simulink model "combined_model_withAC_2023"  (R2023a)
settings: Solver=VariableStepAuto  StartTime=0.0  StopTime=5  RelTol=1e-3
model workspace (MAT data in the model file):
  C = 0.00044
  L = 0.00025
undefined symbols (not defined in the file): C_phi, Ls, poles, R_load, Rs
libraries: spsDiodeLib x7, spsSeriesRLCBranchLib x6, spsVoltageMeasurementLib x5, spsMosfetLib x5, spsControlledVoltageSourceLib x3, simulink x3, spsCurrentMeasurementLib x2, spsParallelRLCBranchLib x2, spsGroundLib x1, spsParallelRLCLoadLib x1, spsVariableCapacitorLib x1, spspowerguiLib x1
settings Model: Creator=maarten  LastModifiedBy=maarten

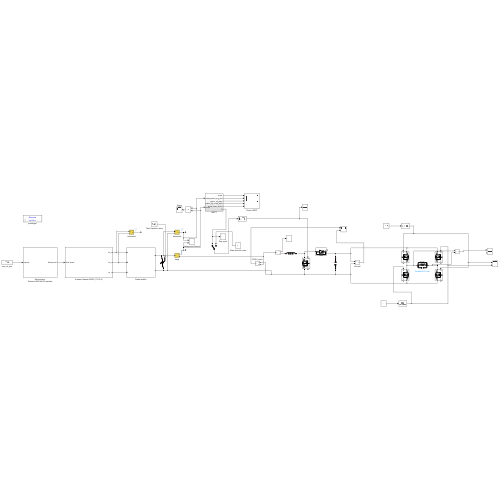
[thumbnail: Simulink's stored preview of the top-level diagram]
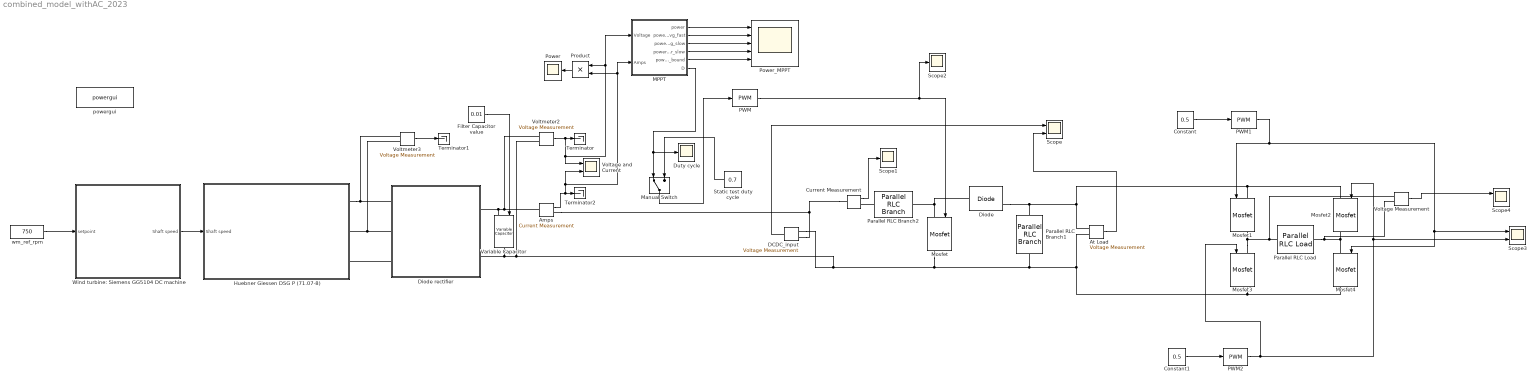
== system combined_model_withAC_2023 ==
  Amps : spsCurrentMeasurementLib/Current Measurement  PhasorSimulation=off  OutputType=Complex  PSBequivalent=0
  At Load : spsVoltageMeasurementLib/Voltage Measurement  PhasorSimulation=off  OutputType=Complex  PSBequivalent=0
  Constant : Constant  Value=0.5
  Constant1 : Constant  Value=0.5
  Current Measurement : spsCurrentMeasurementLib/Current Measurement  PhasorSimulation=off  OutputType=Complex  PSBequivalent=0
  DCDC_input : spsVoltageMeasurementLib/Voltage Measurement  PhasorSimulation=off  OutputType=Complex  PSBequivalent=0
  Diode : spsDiodeLib/Diode  Ron=0.001  Lon=0  Vf=0.8  IC=0  UseSnubber=0  Rs=500  Cs=250e-9  Measurements=on
  Diode rectifier : Subsystem
  Duty cycle : Scope
  Filter Capacitor value : Constant  Value=0.01
  "Huebner Giessen DSG P (71.07-8) " : Subsystem
  MPPT : Subsystem
  Manual Switch : ManualSwitch
  Mosfet{,1..4} (5 alike) : spsMosfetLib/Mosfet  Ron=0.1  Lon=0  Rd=0.01  Vfd=0  IC=0  Rs=1e5  Cs=inf  Measurements=on
  PWM : simulink/Discontinuities/PWM  DisableCoverage=on  Period=0.0001  InitialDelay=0  DisallowZeroDutyCycle=off  RunAtFixedTimeIntervals=off  SampleTime=0.1
  PWM1 : simulink/Discontinuities/PWM  DisableCoverage=on  Period=0.0005  InitialDelay=0  DisallowZeroDutyCycle=off  RunAtFixedTimeIntervals=off  SampleTime=0.1
  PWM2 : simulink/Discontinuities/PWM  DisableCoverage=on  Period=0.0005  InitialDelay=0.0005/2  DisallowZeroDutyCycle=off  RunAtFixedTimeIntervals=off  SampleTime=0.1
  Parallel RLC Branch1 : spsParallelRLCBranchLib/Parallel RLC Branch  LConnTagsString=a  RConnTagsString=__new0  BranchType=C  Resistance=R_load  Inductance=1e-3  SetiL0=off  InitialCurrent=0  Capacitance=C  Setx0=off  InitialVoltage=0  Measurements=None
  Parallel RLC Branch2 : spsParallelRLCBranchLib/Parallel RLC Branch  LConnTagsString=a  RConnTagsString=__new0  BranchType=L  Resistance=R_load  Inductance=L  SetiL0=off  InitialCurrent=0  Capacitance=C  Setx0=off  InitialVoltage=0  Measurements=None
  Parallel RLC Load : spsParallelRLCLoadLib/Parallel RLC Load  LConnTagsString=a  RConnTagsString=__new0  NominalVoltage=1000  NominalFrequency=60  ActivePower=10e3  InductivePower=100  CapacitivePower=100  Setx0=off  InitialVoltage=0  SetiL0=off  InitialCurrent=0  Measurements=None  LoadType=constant Z
      settings: AttributesFormatString=\n  LibrarySourceBlock=sps_lib/Passives/Parallel RLC Load
  Power : Scope
  Power_MPPT : Scope  NumInputPorts=5
  Product : Product
  Scope : Scope  NumInputPorts=2
  Scope1 : Scope
  Scope2 : Scope
  Scope3 : Scope  NumInputPorts=2
  Scope4 : Scope  NumInputPorts=2
  Static test duty cycle : Constant  Value=0.7
  Terminator : Terminator
  Terminator1 : Terminator
  Terminator2 : Terminator
  Variable Capacitor : spsVariableCapacitorLib/Variable Capacitor  methode=Backward Euler  Cabsmin=1e-9  Initialize=off  vC0=0  C0=1e-6  iC0=0
      settings: LibrarySourceBlock=sps_lib/Passives/Variable Capacitor
  Voltage Measurement : spsVoltageMeasurementLib/Voltage Measurement  PhasorSimulation=off  OutputType=Complex  PSBequivalent=0
  Voltage and Current : Scope  NumInputPorts=2
  Voltmeter2 : spsVoltageMeasurementLib/Voltage Measurement  PhasorSimulation=off  OutputType=Complex  PSBequivalent=0
  Voltmeter3 : spsVoltageMeasurementLib/Voltage Measurement  PhasorSimulation=off  OutputType=Complex  PSBequivalent=0
  "Wind turbine: Siemens GG5104 DC machine " : Subsystem
  powergui : spspowerguiLib/powergui  Priority=1  SimulationMode=Discrete  SampleTime=1e-6  frequency=60  Iterations=50  frequencyindice=0  Pbase=100e6  ErrMax=1e-4  UnitsV=kV  UnitsW=MW  buscounter=0  FunctionMessages=off  echomessages=off  EnableUseOfTLC=off  CurrentSourceSwitches=off  DisableSnubberDevices=off  DisableRonSwitches=off  DisableVfSwitches=off  DisplayEquations=off  AutomaticDiscreteSolvers=off  SolverType=Tustin  Interpol=off  ExternalGateDelay=off  methode=off  Ts=0  x0status=blocks  SPID=off  SwTol=0  HookPort=off  NonlinearTolerance=1e-4  nMaxIteration=100  ContinueOnMaxIteration=off  RestoreLinks=warning  ResistiveCurrentMeasurement=off  Frange=[0:2:500]  Ylog=off  Xlog=on  ShowGrid=off  save=off  variable=ZData  structure=0  ZoomFFT=off  StartTime=0.0  cycles=1  DisplayStyle=1  fundamental=60  FreqAxis=off  MaxFrequency=1000  frequencyindicesteady=1  RmsSteady=1  display=off
  wm_ref_rpm : Constant  Value=750
  wires:
  MPPT/2(power_avg_fast) -> Power_MPPT/2
  MPPT/6(D) -> Manual Switch/1, Duty cycle/1
  PWM/1 -> Mosfet/1, Scope2/1
  "Wind turbine: Siemens GG5104 DC machine "/1(Shaft speed) -> "Huebner Giessen DSG P (71.07-8) "/1(Shaft speed)
  wm_ref_rpm/1 -> "Wind turbine: Siemens GG5104 DC machine "/1(setpoint)
  Static test duty cycle/1 -> Manual Switch/2
  Filter Capacitor value/1 -> Variable Capacitor/1
  MPPT/5(power_lower_bound) -> Power_MPPT/5
  MPPT/3(power_avg_slow) -> Power_MPPT/3
  MPPT/4(power_avg_super_slow) -> Power_MPPT/4
  Product/1 -> Power/1
  MPPT/1(power) -> Power_MPPT/1
  Amps/1 -> Voltage and Current/2, Product/2, MPPT/2(Amps), Terminator2/1
  At Load/1 -> Scope/2
  Voltmeter3/1 -> Terminator1/1
  DCDC_input/1 -> Scope/1
  Voltmeter2/1 -> MPPT/1(Voltage), Product/1, Voltage and Current/1, Terminator/1
  Manual Switch/1 -> PWM/1
  Current Measurement/1 -> Scope1/1
  Voltage Measurement/1 -> Scope4/1
  Constant1/1 -> PWM2/1
  Constant/1 -> PWM1/1
  PWM2/1 -> Mosfet3/1, Scope3/2, Mosfet2/1
  PWM1/1 -> Scope3/1, Mosfet4/1, Mosfet1/1
  connections:
  Mosfet3/RConn1 -- Variable Capacitor/RConn1 -- Diode rectifier/RConn2 -- Voltmeter2/LConn2 -- DCDC_input/LConn2 -- Mosfet/RConn1 -- Parallel RLC Branch1/RConn1 -- At Load/LConn2 -- Mosfet4/RConn1
  Mosfet/LConn1 -- Diode/LConn1 -- Parallel RLC Branch2/RConn1
  Mosfet1/LConn1 -- Diode/RConn1 -- Parallel RLC Branch1/LConn1 -- At Load/LConn1 -- Mosfet2/LConn1
  Amps/LConn1 -- Diode rectifier/RConn1 -- Variable Capacitor/LConn1 -- Voltmeter2/LConn1
  Voltmeter3/LConn2 -- "Huebner Giessen DSG P (71.07-8) "/RConn2 -- Diode rectifier/LConn2
  Current Measurement/LConn1 -- DCDC_input/LConn1 -- Amps/RConn1
  Voltmeter3/LConn1 -- Diode rectifier/LConn1 -- "Huebner Giessen DSG P (71.07-8) "/RConn1
  Diode rectifier/LConn3 -- "Huebner Giessen DSG P (71.07-8) "/RConn3
  Parallel RLC Branch2/LConn1 -- Current Measurement/RConn1
  Parallel RLC Load/RConn1 -- Voltage Measurement/LConn2 -- Mosfet4/LConn1 -- Mosfet2/RConn1
  Mosfet3/LConn1 -- Voltage Measurement/LConn1 -- Parallel RLC Load/LConn1 -- Mosfet1/RConn1

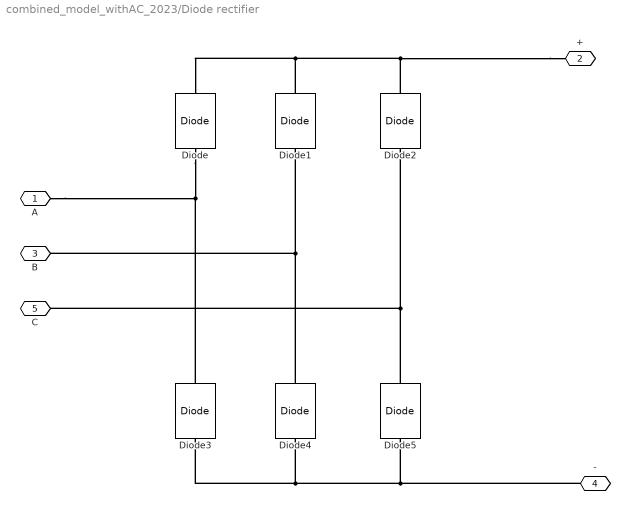
== system combined_model_withAC_2023/Diode rectifier ==
  Diode{,1..5} (6 alike) : spsDiodeLib/Diode  Ron=0.01  Lon=0  Vf=0.85  IC=0  UseSnubber=off  Rs=500  Cs=250e-9  Measurements=off
  A : PMIOPort  Side=Left
  + : PMIOPort  Port=2  Side=Right
  B : PMIOPort  Port=3  Side=Left
  - : PMIOPort  Port=4  Side=Right
  C : PMIOPort  Port=5  Side=Left
  connections:
  Diode2/LConn1 -- C/RConn1 -- Diode5/RConn1
  +/RConn1 -- Diode2/RConn1 -- Diode1/RConn1 -- Diode/RConn1
  Diode3/LConn1 -- -/RConn1 -- Diode5/LConn1 -- Diode4/LConn1
  Diode3/RConn1 -- A/RConn1 -- Diode/LConn1
  Diode1/LConn1 -- B/RConn1 -- Diode4/RConn1

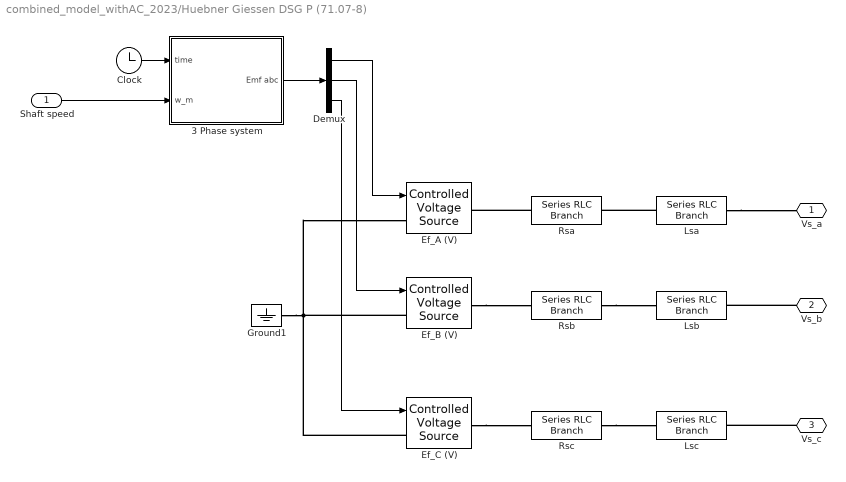
== system combined_model_withAC_2023/Huebner Giessen DSG P (71.07-8)  ==
  Shaft speed : Inport
  "3 Phase system " : Subsystem
  Clock : Clock
  Demux : Demux  Outputs=3
  Ef_A (V) : spsControlledVoltageSourceLib/Controlled Voltage Source  Initialize=on  Source_Type=AC  Amplitude=0  Phase=0  Frequency=0  Measurements=None
  Ef_B (V) : spsControlledVoltageSourceLib/Controlled Voltage Source  Initialize=on  Source_Type=AC  Amplitude=0  Phase=0  Frequency=0  Measurements=None
  Ef_C (V) : spsControlledVoltageSourceLib/Controlled Voltage Source  Initialize=on  Source_Type=AC  Amplitude=0  Phase=0  Frequency=0  Measurements=None
  Ground1 : spsGroundLib/Ground  LConnTagsString=a
  Lsa : spsSeriesRLCBranchLib/Series RLC Branch  LConnTagsString=__new0  RConnTagsString=__new0  BranchType=L  Resistance=Rs  Inductance=Ls  SetiL0=off  InitialCurrent=0  Capacitance=1e-6  Setx0=off  InitialVoltage=0  Measurements=Branch current
  Lsb : spsSeriesRLCBranchLib/Series RLC Branch  LConnTagsString=__new0  RConnTagsString=__new0  BranchType=L  Resistance=Rs  Inductance=Ls  SetiL0=off  InitialCurrent=0  Capacitance=1e-6  Setx0=off  InitialVoltage=0  Measurements=Branch current
  Lsc : spsSeriesRLCBranchLib/Series RLC Branch  LConnTagsString=__new0  RConnTagsString=__new0  BranchType=L  Resistance=Rs  Inductance=Ls  SetiL0=on  InitialCurrent=0  Capacitance=1e-6  Setx0=off  InitialVoltage=0  Measurements=Branch current
  Rsa : spsSeriesRLCBranchLib/Series RLC Branch  LConnTagsString=__new0  RConnTagsString=__new0  BranchType=R  Resistance=Rs  Inductance=Ls  SetiL0=off  InitialCurrent=0  Capacitance=1e-6  Setx0=off  InitialVoltage=0  Measurements=Branch current
  Rsb : spsSeriesRLCBranchLib/Series RLC Branch  LConnTagsString=__new0  RConnTagsString=__new0  BranchType=R  Resistance=Rs  Inductance=Ls  SetiL0=off  InitialCurrent=0  Capacitance=1e-6  Setx0=off  InitialVoltage=0  Measurements=Branch current
  Rsc : spsSeriesRLCBranchLib/Series RLC Branch  LConnTagsString=__new0  RConnTagsString=__new0  BranchType=R  Resistance=Rs  Inductance=Ls  SetiL0=on  InitialCurrent=0  Capacitance=1e-6  Setx0=off  InitialVoltage=0  Measurements=Branch current
  Vs_a : PMIOPort  Side=Right
  Vs_b : PMIOPort  Port=2  Side=Right
  Vs_c : PMIOPort  Port=3  Side=Right
  wires:
  Demux/1 -> Ef_A (V)/1
  Demux/3 -> Ef_C (V)/1
  Demux/2 -> Ef_B (V)/1
  Shaft speed/1 -> "3 Phase system "/2(w_m)
  Clock/1 -> "3 Phase system "/1(time)
  "3 Phase system "/1("Emf abc ") -> Demux/1
  connections:
  Ef_B (V)/RConn1 -- Rsb/LConn1
  Lsa/RConn1 -- Vs_a/RConn1
  Vs_b/RConn1 -- Lsb/RConn1
  Ef_B (V)/LConn1 -- Ground1/LConn1 -- Ef_C (V)/LConn1 -- Ef_A (V)/LConn1
  Vs_c/RConn1 -- Lsc/RConn1
  Lsa/LConn1 -- Rsa/RConn1
  Ef_C (V)/RConn1 -- Rsc/LConn1
  Rsa/LConn1 -- Ef_A (V)/RConn1
  Rsb/RConn1 -- Lsb/LConn1
  Rsc/RConn1 -- Lsc/LConn1

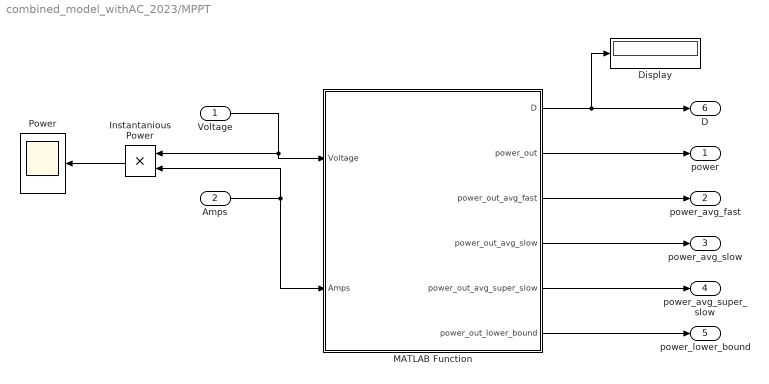
== system combined_model_withAC_2023/MPPT ==
  Voltage : Inport
  Amps : Inport  Port=2
  Display : Display
  Instantanious Power : Product
  MATLAB Function : MATLAB Function  TreatAsAtomicUnit=on  SystemSampleTime=0.0002
  Power : Scope
  power : Outport
  power_avg_fast : Outport  Port=2
  power_avg_slow : Outport  Port=3
  power_avg_super_slow : Outport  Port=4
  power_lower_bound : Outport  Port=5
  D : Outport  Port=6
  wires:
  MATLAB Function/1(D) -> D/1, Display/1
  Instantanious Power/1 -> Power/1
  Voltage/1 -> Instantanious Power/1, MATLAB Function/1(Voltage)
  Amps/1 -> MATLAB Function/2(Amps), Instantanious Power/2
  MATLAB Function/2(power_out) -> power/1
  MATLAB Function/3(power_out_avg_fast) -> power_avg_fast/1
  MATLAB Function/4(power_out_avg_slow) -> power_avg_slow/1
  MATLAB Function/5(power_out_avg_super_slow) -> power_avg_super_slow/1
  MATLAB Function/6(power_out_lower_bound) -> power_lower_bound/1

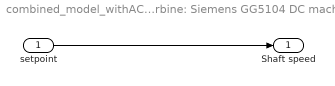
== system combined_model_withAC_2023/Wind turbine: Siemens GG5104 DC machine  ==
  setpoint : Inport
  Shaft speed : Outport
  wires:
  setpoint/1 -> Shaft speed/1

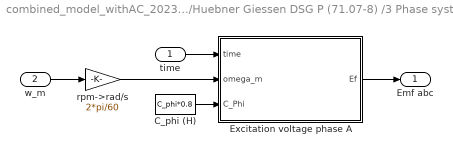
== system combined_model_withAC_2023/Huebner Giessen DSG P (71.07-8) /3 Phase system  ==
  time : Inport
  w_m : Inport  Port=2
  C_phi (H) : Constant  Value=C_phi*0.8  VectorParams1D=off
  Excitation voltage phase A : Subsystem
  rpm->rad/s : Gain  Gain=2*pi/60
  "Emf abc " : Outport
  wires:
  w_m/1 -> rpm->rad/s/1
  C_phi (H)/1 -> Excitation voltage phase A/3(C_Phi)
  time/1 -> Excitation voltage phase A/1(time)
  rpm->rad/s/1 -> Excitation voltage phase A/2(omega_m)
  Excitation voltage phase A/1(Ef) -> "Emf abc "/1

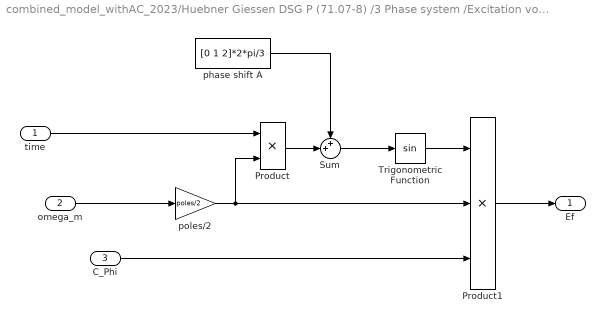
== system combined_model_withAC_2023/Huebner Giessen DSG P (71.07-8) /3 Phase system /Excitation voltage phase A ==
  time : Inport
  omega_m : Inport  Port=2
  C_Phi : Inport  Port=3
  Product : Product  RndMeth=Zero
  Product1 : Product  Inputs=3  RndMeth=Zero
  Sum : Sum  Inputs=++|
  Trigonometric Function : Trigonometry
  phase shift A : Constant  Value=[0 1 2]*2*pi/3
  poles/2 : Gain  Gain=poles/2
  Ef : Outport
  wires:
  poles/2/1 -> Product/2, Product1/2
  Trigonometric Function/1 -> Product1/1
  phase shift A/1 -> Sum/1
  Product/1 -> Sum/2
  Product1/1 -> Ef/1
  C_Phi/1 -> Product1/3
  Sum/1 -> Trigonometric Function/1
  time/1 -> Product/1
  omega_m/1 -> poles/2/1

== matlab function combined_model_withAC_2023/MPPT/MATLAB Function ==
  settings: updateMethod=DISCRETE
  data: Voltage input double; Amps input double; D output double; power_out output double; power_out_avg_fast output; power_out_avg_slow output; power_out_avg_super_slow output; power_out_lower_bound output
function [D, power_out, power_out_avg_fast, power_out_avg_slow, power_out_avg_super_slow, power_out_lower_bound] = fcn(Voltage, Amps)

persistent timeout D_previous direction_previous fast_power_average super_slow_power_average slow_power_average power_lower_bound slow_power_array super_slow_power_array fast_power_array setfast setslow; %counter power_previous 
step_size = 0.0005;
super_slow_filter_size = 5000;
slow_filter_size = 500;
fast_filter_size = 100;
lower_bound_value = 0.95;


if isempty(D_previous)
    setfast = 0;
    timeout = 0;
    setslow = 0;
    D_previous = 0.9;
    direction_previous = 0;
    super_slow_power_array = zeros(super_slow_filter_size,1);
    slow_power_array = zeros(slow_filter_size,1);
    fast_power_array = zeros(fast_filter_size,1);
end

super_slow_power_array(2:end) = super_slow_power_array(1:end-1);
slow_power_array(2:end) = slow_power_array(1:end-1);
fast_power_array(2:end) = fast_power_array(1:end-1);



power = Voltage * Amps;
super_slow_power_array(1) = power;
slow_power_array(1) = power;
fast_power_array(1) = power;

super_slow_power_average = mean(super_slow_power_array);
slow_power_average = mean(slow_power_array);
fast_power_average = mean(fast_power_array);
power_lower_bound = lower_bound_value * super_slow_power_average;
direction = direction_previous;

if slow_power_average > fast_power_average && setfast == 0
    setfast = 1;
    if direction_previous == 1
        direction = 0;
    else
        direction = 1;
    end
end

if power_lower_bound < fast_power_average
    timeout = timeout + 1;
end

%if power_lower_bound > fast_power_average && setslow == 0 && timeout > 100
%    setslow = 1;
%    timeout = 0;
%    if direction_previous == 1
%        direction = 0;
%    else
%        direction = 1;
%    end
%end

if power_lower_bound < fast_power_average
    setslow = 0;
end

if slow_power_average < fast_power_average
    setfast = 0;
end

D = D_previous + (1.213-D_previous) * ((step_size * direction) - (step_size * (1 - direction)));

D_previous = D;
power_out_avg_slow = slow_power_average;
power_out = power;
power_out_avg_fast = fast_power_average;
power_out_avg_super_slow = super_slow_power_average;
power_out_lower_bound = power_lower_bound;
direction_previous = direction;
